simulink model "Lab5_3"  (R2021a)
settings: Solver=VariableStepAuto  StartTime=0.0  StopTime=1000  RelTol=1e-3
values from neighbouring files (symbols this model uses):
  ds_des = 1    [LAB_3.m]
  J = 1.7    [LAB_3.m]
  K = diag([1,1,1,10,10,10])    [LAB_3.m]
  K_phi = diag([1,1,1])    [LAB_3.m]
  k_w = 3    [LAB_3.m]
  m = 2.3    [LAB_3.m]
  pos_init = [-10;-4;10]    [LAB_3.m]
  rot_des = axang2rotm([n_des / norm(n_des) , norm(n_des)])    [LAB_3.m]
  rot_init = axang2rotm([n_init / norm(n_init) , norm(n_init)])    [LAB_3.m]
settings Model: Creator=zein  LastModifiedBy=zein
settings DebuggingCC: UnconnectedInputMsg=none  UnconnectedOutputMsg=none  UnconnectedLineMsg=none
settings ModelReferenceCC: EnableRefExpFcnMdlSchedulingChecks=off
settings RTWCC: Description=Generic Real-Time Target  DLArmComputeVersion=20.02.1

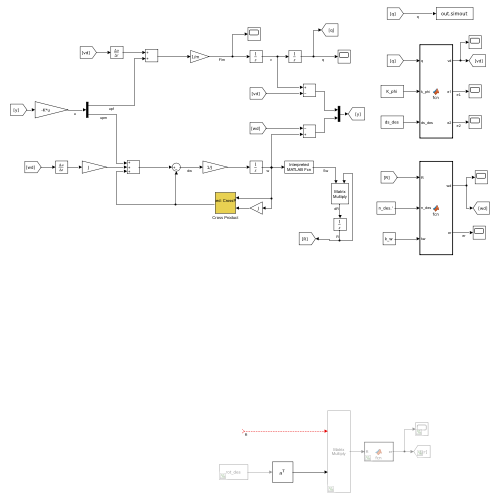
[thumbnail: Simulink's stored preview of the top-level diagram]
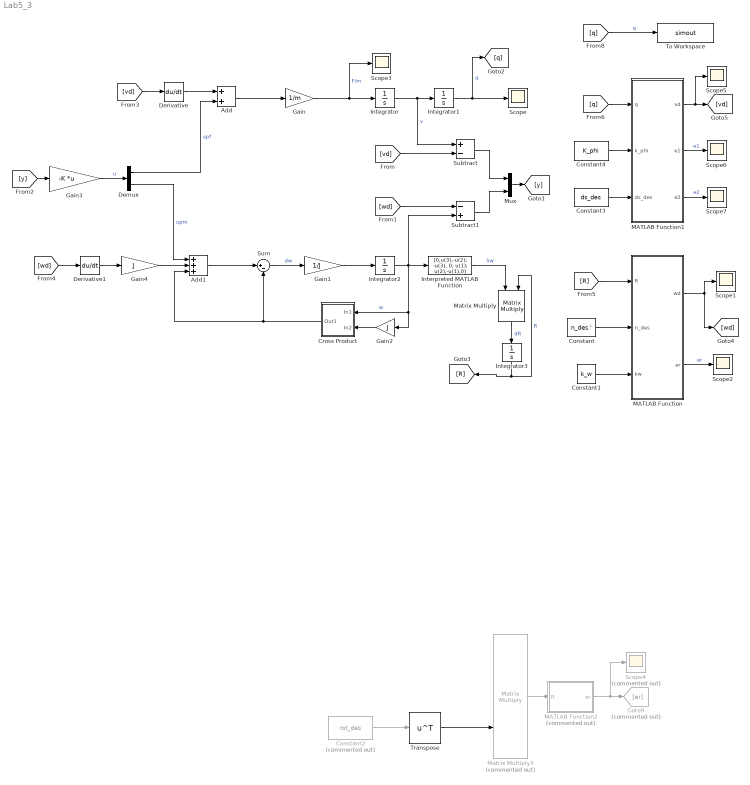
== system Lab5_3 ==
  Add : Sum
  Add1 : Sum  Inputs=+++
  Constant : Constant  Value=n_des.'  VectorParams1D=off
  Constant1 : Constant  Value=k_w
  Constant2 : Constant  Commented=on  Value=rot_des  VectorParams1D=off
  Constant3 : Constant  Value=ds_des
  Constant4 : Constant  Value=K_phi  VectorParams1D=off
  Cross Product : Subsystem  Description=Replaced Block  mask(Replaced Block){}
      mask help: This block has been replaced with an empty subsystem because it used functionality that is unavailable in Simulink R2021a.
      mask Display: fprintf('Replaced: %s\n','CrossProduct')
  Demux : Demux  Outputs=2
  Derivative : Derivative  CoefficientInTFapproximation=10
  Derivative1 : Derivative
  Gain : Gain  Gain=1/m
  Gain1 : Gain  Gain=1/J
  Gain2 : Gain  Gain=J
  Gain3 : Gain  Gain=-K  Multiplication=Matrix(K*u)
  Gain4 : Gain  Gain=J
  Goto9 : Goto  Commented=on  GotoTag=er
  Integrator : Integrator  InitialCondition=[0;0;0]
  Integrator1 : Integrator  InitialCondition=pos_init
  Integrator2 : Integrator  InitialCondition=[0;0;0]
  Integrator3 : Integrator  InitialCondition=rot_init
  Interpreted MATLAB Function : MATLABFcn  MATLABFcn=[0,u(3),-u(2); -u(3), 0, u(1); u(2),-u(1),0]  Output1D=off
  MATLAB Function : MATLAB Function  TreatAsAtomicUnit=on
  MATLAB Function1 : MATLAB Function  TreatAsAtomicUnit=on
  MATLAB Function2 : MATLAB Function  Commented=on  TreatAsAtomicUnit=on
  Matrix Multiply : Product  Multiplication=Matrix(*)
  Matrix Multiply3 : Product  Commented=on  Multiplication=Matrix(*)
  Mux : Mux  Inputs=2
  Scope{,1..3,5..7} (7 alike) : Scope
  Scope4 : Scope  Commented=on
  Subtract : Sum  Inputs=+-
  Subtract1 : Sum  Inputs=-+
  Sum : Sum  Inputs=|+-
  To Workspace : ToWorkspace  VariableName=simout  SaveFormat=Timeseries  SampleTime=-1
  Transpose : Math  Operator=transpose  SaturateOnIntegerOverflow=on
  wires:
  Integrator/1 -> Subtract/1, Integrator1/1  "v"
  Gain/1 -> Scope3/1, Integrator/1  "F/m"
  Integrator1/1 -> [q], Scope/1  "q"
  [vd] -> Subtract/2
  Gain2/1 -> Cross Product/2(In2)
  Integrator2/1 -> Subtract1/2, Gain2/1, Cross Product/1(In1), Interpreted MATLAB Function/1  "w"
  Gain1/1 -> Integrator2/1
  Sum/1 -> Gain1/1  "dw"
  Cross Product/1(Out1) -> Add1/3, Sum/2
  [wd] -> Subtract1/1
  Subtract/1 -> Mux/1
  Subtract1/1 -> Mux/2
  Mux/1 -> [y]
  [y] -> Gain3/1
  Gain3/1 -> Demux/1  "u"
  Add/1 -> Gain/1
  Add1/1 -> Sum/1
  [vd] -> Derivative/1
  Derivative/1 -> Add/1
  Demux/1 -> Add/2  "upf"
  Gain4/1 -> Add1/2
  [wd] -> Derivative1/1
  Derivative1/1 -> Gain4/1
  Demux/2 -> Add1/1  "upm"
  Integrator3/1 -> Matrix Multiply/2, [R]  "R"
  Matrix Multiply/1 -> Integrator3/1  "dR"
  Interpreted MATLAB Function/1 -> Matrix Multiply/1  "Sw"
  Constant/1 -> MATLAB Function/2(n_des)
  Constant1/1 -> MATLAB Function/3(kw)
  [R] -> MATLAB Function/1(R)
  MATLAB Function/1(wd) -> [wd], Scope1/1
  MATLAB Function/2(er) -> Scope2/1  "er"
  MATLAB Function2/1(er) -> Scope4/1, Goto9/1
  Transpose/1 -> Matrix Multiply3/2
  ? -> Matrix Multiply3/1  "R"
  Matrix Multiply3/1 -> MATLAB Function2/1(R)
  Constant2/1 -> Transpose/1
  Constant3/1 -> MATLAB Function1/3(ds_des)
  Constant4/1 -> MATLAB Function1/2(k_phi)
  [q] -> MATLAB Function1/1(q)
  MATLAB Function1/1(vd) -> Scope5/1, [vd]
  MATLAB Function1/2(e1) -> Scope6/1  "e1"
  MATLAB Function1/3(e2) -> Scope7/1  "e2"
  [q] -> To Workspace/1  "q"

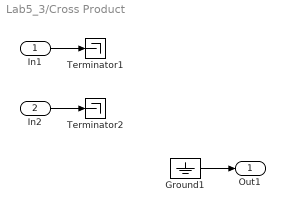
== system Lab5_3/Cross Product ==
  In1 : Inport
  In2 : Inport  Port=2
  Ground1 : Ground
  Terminator1 : Terminator
  Terminator2 : Terminator
  Out1 : Outport
  wires:
  Ground1/1 -> Out1/1
  In2/1 -> Terminator2/1
  In1/1 -> Terminator1/1

== matlab function Lab5_3/MATLAB Function1 ==
  data: q input; k_phi input; vd output; ds_des input; e1 output; e2 output
function [vd,e1,e2]  = fcn(q,k_phi,ds_des)

x = q(1);
y = q(2);
z = q(3);

u_phi = - k_phi * [x.*(x.^2+y.^2-4.0e+2).*2.0;y+z+y.*(x.^2+y.^2-4.0e+2).*2.0-1.0e+1;y+z-1.0e+1];

J = [[y.*1.0./sqrt(x.^2.*2.0+y.^2);x.*1.0./sqrt(x.^2+y.^2);0.0], ...
     [-x.*1.0./sqrt(x.^2.*2.0+y.^2);y.*1.0./sqrt(x.^2+y.^2);sqrt(2.0)./2.0],...
     [x.*1.0./sqrt(x.^2.*2.0+y.^2);0.0;sqrt(2.0)./2.0]];

u_tau = (J^-1) * [ds_des;0;0];

vd = u_tau + u_phi;

e1 = x^2 +y^2 -400;
e2 = z+y-10;

== matlab function Lab5_3/MATLAB Function ==
  data: R input; n_des input; wd output; kw input; er output
function [wd, er] = fcn(R, n_des, kw)

n = rotm2axang(R);
n = n(1:3)*n(4);
n = n.';


Sc = [0,n_des(3),-n_des(2); -n_des(3), 0, n_des(1); n_des(2),-n_des(1),0];

wd = -Sc * n * kw * (1-n.'*n_des);
er = (1-n.'*n_des);
% wd = 0

== matlab function Lab5_3/MATLAB Function2 ==
  data: R input; er output
function er = fcn(R)

A = R - R.';

e = [A(2,3); A(3,1); A(1,2)];

er = e/2;
